simulink model "lqr_c"  (R2018a)
settings: Solver=VariableStepAuto  StartTime=0.0  StopTime=Tmax  FixedStep=1/Ts  RelTol=1e-3
values from neighbouring files (symbols this model uses):
  Lw = [c_tilt*c_angle -c_tilt*s_angle -c_tilt*c_angle  c_tilt*s_angle ... (first row only)    [get_transformation_matrix.m]
undefined symbols (not defined in the file or in its folder): des_phi, des_psi, des_theta, I_motor, I_wheel, init_phi, init_psi, init_theta, Ip, K_lqr, Kt, Kv, omega_i_x, omega_i_y, omega_i_z, T_ext_x, T_ext_y, T_ext_z
libraries: simulink_extras x5, sharedutil x2, dspmtrx3 x1
settings Model: Creator=Renz  LastModifiedBy=Renz

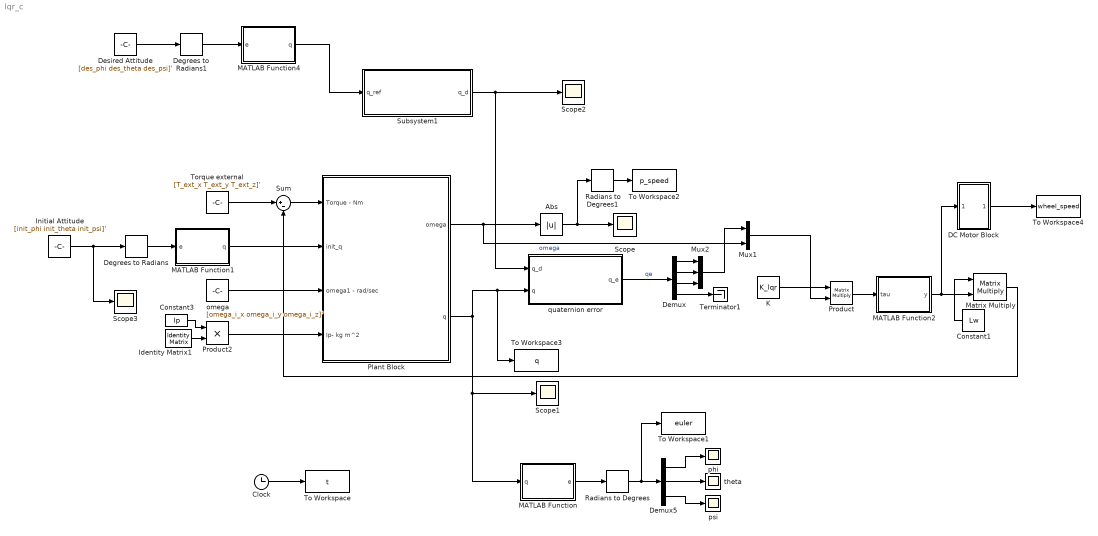
== system lqr_c ==
  Abs : Abs
  Clock : Clock
  Constant1 : Constant  Value=Lw
  Constant3 : Constant  Value=Ip
  DC Motor Block : Subsystem
  Degrees to Radians : simulink_extras/Transformations/Degrees to Radians
  Degrees to Radians1 : simulink_extras/Transformations/Degrees to Radians
  Demux : Demux
  Demux5 : Demux  Outputs=3
  Desired Attitude : Constant  Value=[des_phi des_theta des_psi]'
  Identity Matrix1 : dspmtrx3/Identity Matrix  Inherit=off  N=3  Ts=1  dataType=double  isSigned=on  wordLen=16  udDataType=sfix(16)  fracBitsMode=Best precision  numFracBits=15  OutDataTypeStr=double  LastOutDataTypeStr=double
      settings: SourceProductName=DSP System Toolbox
  Initial Attitude : Constant  Value=[init_phi init_theta init_psi]'
  K : Constant  Value=K_lqr
  MATLAB Function : MATLAB Function  TreatAsAtomicUnit=on
  MATLAB Function1 : MATLAB Function  TreatAsAtomicUnit=on
  MATLAB Function2 : MATLAB Function  TreatAsAtomicUnit=on
  MATLAB Function4 : MATLAB Function  TreatAsAtomicUnit=on
  Matrix Multiply : Product  Multiplication=Matrix(*)
  Mux1 : Mux  Inputs=2
  Mux2 : Mux  Inputs=3
  Plant Block : Subsystem
  Product : Product  Multiplication=Matrix(*)
  Product2 : Product
  Radians to Degrees : simulink_extras/Transformations/Radians to Degrees
  Radians to Degrees1 : simulink_extras/Transformations/Radians to Degrees
  Scope{,1..3} (4 alike) : Scope
  Subsystem1 : Subsystem
  Sum : Sum  Inputs=|+-
  Terminator1 : Terminator
  To Workspace : ToWorkspace  VariableName=t  SampleTime=-1
  To Workspace1 : ToWorkspace  VariableName=euler  SampleTime=-1
  To Workspace2 : ToWorkspace  VariableName=p_speed  SampleTime=-1
  To Workspace3 : ToWorkspace  VariableName=q  SampleTime=-1
  To Workspace4 : ToWorkspace  VariableName=wheel_speed  SampleTime=-1
  Torque external : Constant  Value=[T_ext_x T_ext_y T_ext_z]'
  omega : Constant  Value=[omega_i_x omega_i_y omega_i_z]'
  phi : Scope
  psi : Scope
  quaternion error : Subsystem
  theta : Scope
  wires:
  MATLAB Function/1(e) -> Radians to Degrees/1
  Degrees to Radians/1 -> MATLAB Function1/1(e)
  Demux5/2 -> theta/1
  Plant Block/2(q) -> To Workspace3/1, quaternion error/2(q), MATLAB Function/1(q), Scope1/1
  Subsystem1/1(q_d) -> quaternion error/1(q_d), Scope2/1
  Demux5/1 -> phi/1
  Sum/1 -> Plant Block/1(Torque - Nm)
  MATLAB Function4/1(q) -> Subsystem1/1(q_ref)
  Constant3/1 -> Product2/1
  MATLAB Function1/1(q) -> Plant Block/2(init_q)
  Torque external/1 -> Sum/1
  Clock/1 -> To Workspace/1
  quaternion error/1(q_e) -> Demux/1  "qe"
  omega/1 -> Plant Block/3(omega1 - rad/sec)
  Plant Block/1(omega) -> Abs/1, Mux1/2  "omega"
  Radians to Degrees/1 -> To Workspace1/1, Demux5/1
  Product2/1 -> Plant Block/4(Ip- kg m^2)
  Identity Matrix1/1 -> Product2/2
  Demux5/3 -> psi/1
  MATLAB Function2/1(y) -> Matrix Multiply/2, DC Motor Block/1(In1)
  Mux1/1 -> Product/2
  Abs/1 -> Scope/1, Radians to Degrees1/1
  Product/1 -> MATLAB Function2/1(tau)
  Matrix Multiply/1 -> Sum/2
  Demux/2 -> Mux2/2
  Demux/1 -> Mux2/1
  Demux/3 -> Mux2/3
  Mux2/1 -> Mux1/1
  K/1 -> Product/1
  Demux/4 -> Terminator1/1
  Initial Attitude/1 -> Scope3/1, Degrees to Radians/1
  Degrees to Radians1/1 -> MATLAB Function4/1(e)
  Desired Attitude/1 -> Degrees to Radians1/1
  Constant1/1 -> Matrix Multiply/1
  DC Motor Block/1(Out1) -> To Workspace4/1
  Radians to Degrees1/1 -> To Workspace2/1

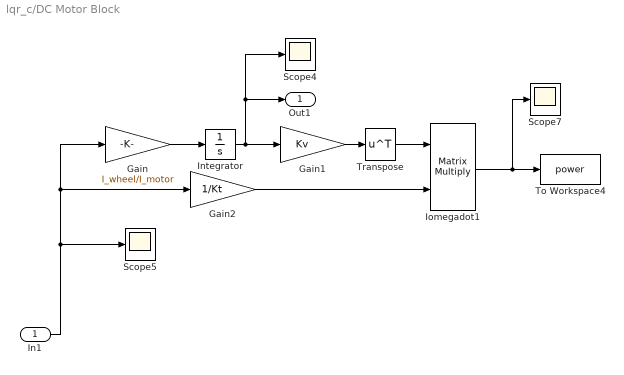
== system lqr_c/DC Motor Block ==
  In1 : Inport
  Gain : Gain  Gain=I_wheel/I_motor
  Gain1 : Gain  Gain=Kv
  Gain2 : Gain  Gain=1/Kt
  Integrator : Integrator
  Iomegadot1 : Product  Multiplication=Matrix(*)
  Scope4 : Scope
  Scope5 : Scope
  Scope7 : Scope
  To Workspace4 : ToWorkspace  VariableName=power  SampleTime=-1
  Transpose : Math  Operator=transpose  SaturateOnIntegerOverflow=on
  Out1 : Outport
  wires:
  Gain/1 -> Integrator/1
  Gain2/1 -> Iomegadot1/2
  Iomegadot1/1 -> Scope7/1, To Workspace4/1
  Transpose/1 -> Iomegadot1/1
  In1/1 -> Scope5/1, Gain2/1, Gain/1
  Integrator/1 -> Out1/1, Scope4/1, Gain1/1
  Gain1/1 -> Transpose/1

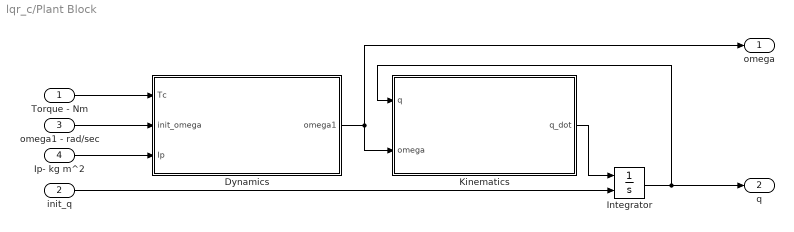
== system lqr_c/Plant Block ==
  Torque - Nm : Inport
  init_q : Inport  Port=2
  omega1 - rad/sec : Inport  Port=3
  Ip- kg m^2 : Inport  Port=4
  Dynamics : Subsystem
  Integrator : Integrator  InitialConditionSource=external
  Kinematics : Subsystem
  omega : Outport
  q : Outport  Port=2
  wires:
  Kinematics/1(q_dot) -> Integrator/1
  Integrator/1 -> Kinematics/1(q), q/1
  Torque - Nm/1 -> Dynamics/1(Tc)
  omega1 - rad/sec/1 -> Dynamics/2(init_omega)
  init_q/1 -> Integrator/2
  Dynamics/1(omega1) -> Kinematics/2(omega), omega/1
  Ip- kg m^2/1 -> Dynamics/3(Ip)

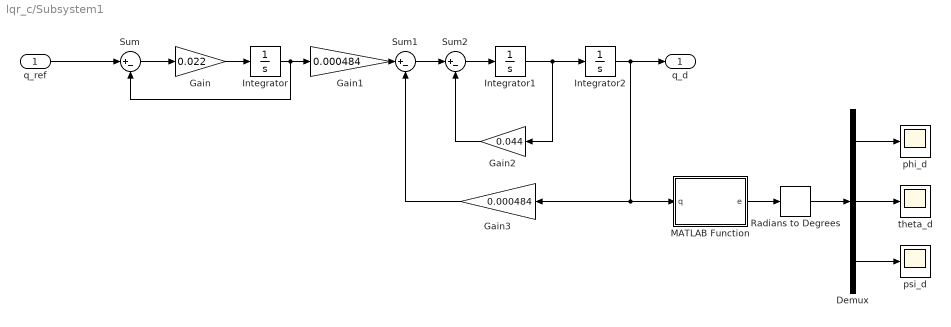
== system lqr_c/Subsystem1 ==
  q_ref : Inport
  Demux : Demux  Outputs=3
  Gain : Gain  Gain=0.022
  Gain1 : Gain  Gain=0.000484
  Gain2 : Gain  Gain=0.044
  Gain3 : Gain  Gain=0.000484
  Integrator : Integrator
  Integrator1 : Integrator
  Integrator2 : Integrator
  MATLAB Function : MATLAB Function  TreatAsAtomicUnit=on
  Radians to Degrees : simulink_extras/Transformations/Radians to Degrees
  Sum : Sum  Inputs=|+-
  Sum1 : Sum  Inputs=|+-
  Sum2 : Sum  Inputs=|+-
  phi_d : Scope
  psi_d : Scope
  theta_d : Scope
  q_d : Outport
  wires:
  Demux/3 -> psi_d/1
  Gain1/1 -> Sum1/1
  Sum/1 -> Gain/1
  Gain2/1 -> Sum2/2
  Demux/2 -> theta_d/1
  Gain/1 -> Integrator/1
  Integrator/1 -> Gain1/1, Sum/2
  Sum1/1 -> Sum2/1
  Gain3/1 -> Sum1/2
  Integrator1/1 -> Gain2/1, Integrator2/1
  Sum2/1 -> Integrator1/1
  q_ref/1 -> Sum/1
  Demux/1 -> phi_d/1
  Radians to Degrees/1 -> Demux/1
  Integrator2/1 -> q_d/1, MATLAB Function/1(q), Gain3/1
  MATLAB Function/1(e) -> Radians to Degrees/1

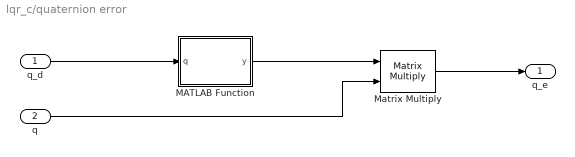
== system lqr_c/quaternion error ==
  q_d : Inport
  q : Inport  Port=2
  MATLAB Function : MATLAB Function  TreatAsAtomicUnit=on
  Matrix Multiply : Product  Multiplication=Matrix(*)
  q_e : Outport
  wires:
  MATLAB Function/1(y) -> Matrix Multiply/1
  Matrix Multiply/1 -> q_e/1
  q/1 -> Matrix Multiply/2
  q_d/1 -> MATLAB Function/1(q)

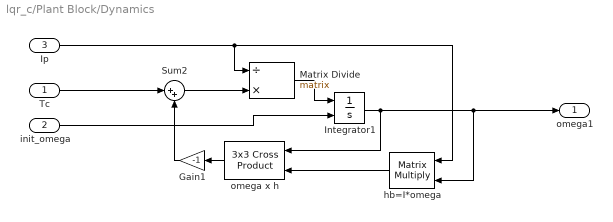
== system lqr_c/Plant Block/Dynamics ==
  Tc : Inport
  init_omega : Inport  Port=2
  Ip : Inport  Port=3
  Gain1 : Gain  Gain=-1
  Integrator1 : Integrator  InitialConditionSource=external  ZeroCross=off
  Matrix Divide : Product  Inputs=/*  Multiplication=Matrix(*)
  Sum2 : Sum  Inputs=|++
  hb=I*omega : Product  Multiplication=Matrix(*)
  omega x h : sharedutil/3x3 Cross Product  aMode=aMode
      settings: SourceProductBaseCode=AE
  omega1 : Outport
  wires:
  Gain1/1 -> Sum2/2
  Integrator1/1 -> omega x h/1, omega1/1, hb=I*omega/2
  init_omega/1 -> Integrator1/2
  Sum2/1 -> Matrix Divide/2
  hb=I*omega/1 -> omega x h/2
  omega x h/1 -> Gain1/1
  Tc/1 -> Sum2/1
  Matrix Divide/1 -> Integrator1/1
  Ip/1 -> Matrix Divide/1, hb=I*omega/1

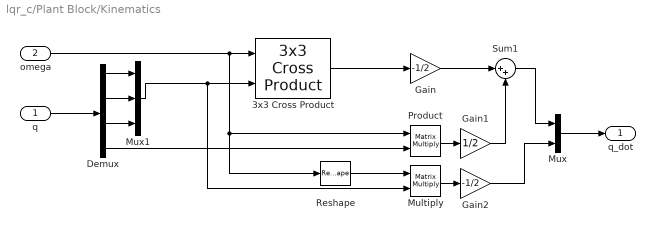
== system lqr_c/Plant Block/Kinematics ==
  q : Inport
  omega : Inport  Port=2
  3x3 Cross Product : sharedutil/3x3 Cross Product  aMode=aMode
      settings: SourceProductBaseCode=AE
  Demux : Demux
  Gain : Gain  Gain=-1/2
  Gain1 : Gain  Gain=1/2
  Gain2 : Gain  Gain=-1/2
  Multiply : Product  Multiplication=Matrix(*)
  Mux : Mux  Inputs=2
  Mux1 : Mux  Inputs=3
  Product : Product  Multiplication=Matrix(*)
  Reshape : Reshape  OutputDimensionality=Row vector (2-D)
  Sum1 : Sum  Inputs=|++
  q_dot : Outport
  wires:
  omega/1 -> 3x3 Cross Product/1, Product/1, Reshape/1
  Mux1/1 -> Multiply/2, 3x3 Cross Product/2
  Gain1/1 -> Sum1/2
  3x3 Cross Product/1 -> Gain/1
  Product/1 -> Gain1/1
  Multiply/1 -> Gain2/1
  Gain/1 -> Sum1/1
  Demux/4 -> Product/2
  Sum1/1 -> Mux/1
  Gain2/1 -> Mux/2
  Reshape/1 -> Multiply/1
  Mux/1 -> q_dot/1
  Demux/1 -> Mux1/1
  q/1 -> Demux/1
  Demux/2 -> Mux1/2
  Demux/3 -> Mux1/3

== matlab function lqr_c/Subsystem1/MATLAB Function ==
  data: q input; e output
function e = quat2euler(q)

q0 = q(1,:);
q1 = q(2,:);
q2 = q(3,:);
q3 = q(4,:);

phi = atan((2*(q2*q3 + q0*q1))/(q0^2 - q1^2 - q2^2 + q3^2)); 
theta = asin(-2*(q1*q3 - q0*q2));
psi = atan((2*(q1*q2 + q0*q3))/(q0^2 + q1^2 -q2^2 - q3^2)); 

e = [phi;theta;psi];

end

== matlab function lqr_c/MATLAB Function4 ==
  data: e input; q output
function q = euler2quat(e)

e1 = 0.5*e(1,:);
e2 = 0.5*e(2,:);
e3 = 0.5*e(3,:);

q0 = (sin(e1)*sin(e2)*sin(e3)) + (cos(e1)*cos(e2)*cos(e3));
q1 = (-sin(e2)*sin(e3)*cos(e1)) + (sin(e1)*cos(e2)*cos(e3));
q2 = (sin(e1)*cos(e2)*sin(e3)) + (sin(e2)*cos(e1)*cos(e3));
q3 = (sin(e3)*cos(e1)*cos(e2)) - (sin(e1)*sin(e2)*cos(e3));

q = [q0;q1;q2;q3];

end

== matlab function lqr_c/MATLAB Function1 ==
  data: e input; q output
function q = euler2quat(e)

e1 = 0.5*e(1,:);
e2 = 0.5*e(2,:);
e3 = 0.5*e(3,:);

q0 = (sin(e1)*sin(e2)*sin(e3)) + (cos(e1)*cos(e2)*cos(e3));
q1 = (-sin(e2)*sin(e3)*cos(e1)) + (sin(e1)*cos(e2)*cos(e3));
q2 = (sin(e1)*cos(e2)*sin(e3)) + (sin(e2)*cos(e1)*cos(e3));
q3 = (sin(e3)*cos(e1)*cos(e2)) - (sin(e1)*sin(e2)*cos(e3));

q = [q0;q1;q2;q3];

end

== matlab function lqr_c/quaternion error/MATLAB Function ==
  data: q input; y output
function y = q_error(q)
q1 = q(1,:);
q2 = q(2,:);
q3 = q(3,:);
q4 = q(4,:);

y = [q4,q3,-q2,-q1; -q3,q4,q1,-q2; q2,-q1,q4,-q3; q1,q2,q3,q4];

== matlab function lqr_c/MATLAB Function ==
  data: q input; e output
function e = quat2euler(q)

q0 = q(1,:);
q1 = q(2,:);
q2 = q(3,:);
q3 = q(4,:);

phi = atan((2*(q2*q3 + q0*q1))/(q0^2 - q1^2 - q2^2 + q3^2)); 
theta = asin(-2*(q1*q3 - q0*q2));
psi = atan((2*(q1*q2 + q0*q3))/(q0^2 + q1^2 -q2^2 - q3^2)); 

e = [phi;theta;psi];

end

== matlab function lqr_c/MATLAB Function2 ==
  data: tau input; y output
function y = control_alloc(tau)
K =[1 0 0 0 
    0 1 0 0 
    0 0 1 0 
    0 0 0 1];
T = [0.57735, -0.57735, -0.57735, 0.57735; 0.57735, -0.57735, 0.57735, -0.57735; 0.57735, 0.57735, -0.57735, -0.57735];
W = [1 0 0 0     
    0 1 0 0      
    0 0 1 0      
    0 0 0 1];


y = ucalloc(K,T,W,tau);
